simulink model "Control_test"  (R2014b)
settings: Solver=FixedStepDiscrete  StartTime=0.0  StopTime=Inf  FixedStep=0.001  RelTol=1e-3
PostLoadFcn:
  | , if any(exist('dsrtsu_mdlpostloadfcn', 'file') == [2, 3, 6]), try dsrtsu_mdlpostloadfcn('Execute', bdroot); catch fprintf('Error in PostLoadFcn (dsrtsu_mdlpostloadfcn) for model "%s":\n %s\n', bdroot, lasterr); end, end,
undefined symbols (not defined in the file or in its folder): dtLocal, slcm
libraries: rtican x163, simulink x14
(part 24 of 34)

== system Control_test/InputProcessing/RadarCanProcessing/Track34 ==
  Bus Creator : BusCreator  Inputs=12
  ESR_Track34 : rtican/RTICAN Receive (RX)   Reserved1=[]  Reserved2=[]  Reserved3=[]  Reserved4=[]  SfcnMessage=[]  Msg_Struct=[]  BoardTypeNo=[]  BoardNo=[]  ChannelNo=[]  Parameters=[]  DialogFcn=[]  UnitName=[]  Revision=[]  UnitValues=[]  DSProperties=struct('RTI',struct('Version',uint32(5),'BlockType',struct('isSLSource',uint8(1),'isSLSink',uint8(1),'isHWSource',uint8(0),'isHWSink',uint8(0),'isSetup',uint8(0),'isInline',uint8(1),'isNonInline',uint8(0),'isInterrupt',uint8(0),'isChannelwise',uint8(0)),'IOBoardType','RTICAN','UnitType','MESSAGE','Identifier','RX','DialogType','MSVC','BlockSet','RTICAN','SlaveProcessor','CAN'))  RTIBlockInterface=struct('OutputPortsWidth',int32([1 1 1 1 1 1 1 1 1 1 1 1]),'OutputPortsActive',[1 1 1 1 1 1 1 1 1 1 1 1],'OutputPortsName',{{'CAN_TX_TRACK_RANGE_RATE_34','CAN_TX_TRACK_MED_RANGE_MODE_34','CAN_TX_TRACK_RANGE_ACCEL_34','CAN_TX_TRACK_WIDTH_34','CAN_TX_TRACK_ROLLING_COUNT_34','CAN_TX_TRACK_BRIDGE_OBJECT_34','CAN_TX_TRACK_RANGE_34','CAN_TX_TRACK_ANGLE_34','CAN_TX_TRACK_STATUS_34','CAN_TX_TRACK_ONCOMING_34','CAN_TX_TRACK_GROUPING_CHANGED_34','CAN_TX_TRACK_LAT_RATE_34'}},'OutputPortsDataType',{{'SS_DOUBLE','SS_DOUBLE','SS_DOUBLE','SS_DOUBLE','SS_DOUBLE','SS_DOUBLE','SS_DOUBLE','SS_DOUBLE','SS_DOUBLE','SS_DOUBLE','SS_DOUBLE','SS_DOUBLE'}},'OutputPortsLabel',{{'CAN_TX_TRACK_RANGE_RATE_34','CAN_TX_TRACK_MED_RANGE_MODE_34','CAN_TX_TRACK_RANGE_ACCEL_34','CAN_TX_TRACK_WIDTH_34','CAN_TX_TRACK_ROLLING_COUNT_34','CAN_TX_TRACK_BRIDGE_OBJECT_34','CAN_TX_TRACK_RANGE_34','CAN_TX_TRACK_ANGLE_34','CAN_TX_TRACK_STATUS_34','CAN_TX_TRACK_ONCOMING_34','CAN_TX_TRACK_GROUPING_CHANGED_34','CAN_TX_TRACK_LAT_RATE_34'}},'OutputPortsLabelMode','ON','InputPortsWidth',int32(0),'InputPortsActive',0,'DialogFcn','rtican_message_interface_gui','BlockDisplay',{{'','center'}},'IconTransparency','on','ParameterTunableNames',{{}},'InitLevel',3,'BlockName',struct('Token',{{'ESR_Track34'}}),'SampleTime',{{0.01}},'TriggerPort',{{'none'}},'EnablePort',{{'none'}})  RTIBlockParameters=struct('BoardTypeNo',{{1,'OFF',[]}},'BoardNo',{{2,'ON',[1 16]}},'ChannelNo',{{2,'ON',[1 2]}},'Parameters',{{struct('DataFileSupport',struct('DataFileSelectedMaster',1,'DataFileSelectedLocal',0,'DataFileName','c:\users\mpc_car\documents\github\mpc-car\controller\dbcfiles\esr_dv3_64tgt.dbc|','DataFileDate',{{{['02-Nov-2012 20:32:52']},{['21-Mar-2013 13:39:53']},{['28-Sep-2011 17:08:52']}}},'SelectedFile',['<no file selected>'],'InterfaceFcn','rtican_dbc_file_parser'),'Options',struct('StatusSelected',0,'TimeSelected',0,'DeltaTimeSelected',0,'BytePortSelected',0,'MessageLengthSelected',0,'TriggerPort',struct('Selected',0,'TriggerType',0),'UserCoding',struct('Selected',0,'InterfaceFile','UserDecodingFile','FcnName','UserDecodeFcn','InportSelected',0,'InportWidth',1,'OutportSelected',0,'OutportWidth',1),'EnablePortSelected',0,'SignalOnPortnameSelected',1,'UseRXService',0),'Message',struct('MsgOnBlocknameSelected',1,'MsgName','ESR_Track34','MsgIdFormat',0,'MsgId',1313,'MsgLength',8,'NumSignals',12,'SampleTime',0.01,'Signal',struct('SgnName',{'CAN_TX_TRACK_RANGE_RATE_34','CAN_TX_TRACK_MED_RANGE_MODE_34','CAN_TX_TRACK_RANGE_ACCEL_34','CAN_TX_TRACK_WIDTH_34','CAN_TX_TRACK_ROLLING_COUNT_34','CAN_TX_TRACK_BRIDGE_OBJECT_34','CAN_TX_TRACK_RANGE_34','CAN_TX_TRACK_ANGLE_34','CAN_TX_TRACK_STATUS_34','CAN_TX_TRACK_ONCOMING_34','CAN_TX_TRACK_GROUPING_CHANGED_34','CAN_TX_TRACK_LAT_RATE_34'},'SgnStartBit',{0,14,16,26,30,31,32,43,53,56,57,58},'SgnLength',{14,2,10,4,1,1,11,10,3,1,1,6},'SgnType',{0,0,0,0,0,0,0,0,0,0,0,0},'ModeValue',{-1,-1,-1,-1,-1,-1,-1,-1,-1,-1,-1,-1},'DataType',{1,0,1,0,0,0,0,1,0,0,0,1},'ByteLayout',{2,2,2,2,2,2,2,2,2,2,2,2},'Factor',{0.01,1,0.05,0.5,1,1,0.1,0.1,1,1,1,0.25},'Offset',{0,0,0,0,0,0,0,0,0,0,0,0},'SgnComment',{{''},{''},{''},{''},{''},{''},{''},{''},{''},{''},{''},{''}},'SgnUnit',{'m/s','','m/s/s','m','','','m','deg','','','',''},'Min',{-81.92,0,-25.6,0,0,0,0,-51.2,0,0,0,-8},'Max',{81.91,3,25.55,7.5,1,0,204.7,51.1,7,0,0,7.75},'SLDataType',{'SS_DOUBLE','SS_DOUBLE','SS_DOUBLE','SS_DOUBLE','SS_DOUBLE','SS_DOUBLE','SS_DOUBLE','SS_DOUBLE','SS_DOUBLE','SS_DOUBLE','SS_DOUBLE','SS_DOUBLE'}),'MsgIdNumFormat',0,'MsgComment',{{''}}),'Version',1.2,'general',struct('isFromLib',0)),'OFF',[]}},'GroupId',{{struct('Group',{{'RTICAN'}},'No',4,'Behavior',{{'NAMECHANGE'}},'BlockType',{{'SINK'}},'NameChangeFlag',0),'OFF',[]}},'SFcnRTICANMessage',{{struct('MsgType','RX','SFcnPortType','Scalar','MsgName','ESR_Track34','MsgIdFormat','STD','MsgId',1313,'MsgLength',8,'NumSignals',12,'SampleTime',0.01,'Signal',struct('SgnName',{'CAN_TX_TRACK_RANGE_RATE_34','CAN_TX_TRACK_MED_RANGE_MODE_34','CAN_TX_TRACK_RANGE_ACCEL_34','CAN_TX_TRACK_WIDTH_34','CAN_TX_TRACK_ROLLING_COUNT_34','CAN_TX_TRACK_BRIDGE_OBJECT_34','CAN_TX_TRACK_RANGE_34','CAN_TX_TRACK_ANGLE_34','CAN_TX_TRACK_STATUS_34','CAN_TX_TRACK_ONCOMING_34','CAN_TX_TRACK_GROUPING_CHANGED_34','CAN_TX_TRACK_LAT_RATE_34'},'SgnStartBit',{0,14,16,26,30,31,32,43,53,56,57,58},'SgnLength',{14,2,10,4,1,1,11,10,3,1,1,6},'SgnType',{'standard','standard','standard','standard','standard','standard','standard','standard','standard','standard','standard','standard'},'ModeValue',{-1,-1,-1,-1,-1,-1,-1,-1,-1,-1,-1,-1},'DataType',{['signed int'],['unsigned int'],['signed int'],['unsigned int'],['unsigned int'],['unsigned int'],['unsigned int'],['signed int'],['unsigned int'],['unsigned int'],['unsigned int'],['signed int']},'ByteLayout',{['motorola back.'],['motorola back.'],['motorola back.'],['motorola back.'],['motorola back.'],['motorola back.'],['motorola back.'],['motorola back.'],['motorola back.'],['motorola back.'],['motorola back.'],['motorola back.']},'Factor',{0.01,1,0.05,0.5,1,1,0.1,0.1,1,1,1,0.25},'Offset',{0,0,0,0,0,0,0,0,0,0,0,0},'SLDataType',{'SS_DOUBLE','SS_DOUBLE','SS_DOUBLE','SS_DOUBLE','SS_DOUBLE','SS_DOUBLE','SS_DOUBLE','SS_DOUBLE','SS_DOUBLE','SS_DOUBLE','SS_DOUBLE','SS_DOUBLE'}),'StatusSelected','no','TimeSelected','no','DeltaTimeSelected','no','BytePortSelected','no','MessageLengthSelected','no','TriggerPort',struct('Selected','no','TriggerType',0),'UserCoding',struct('Selected','no','InterfaceFile','UserDecodingFile','FcnName','UserDecodeFcn','InportSelected','no','InportWidth',1,'OutportSelected','no','OutportWidth',1),'EnablePortSelected','no','UseRXService','no','BoardType','DS1','BoardNo',2,'ControllerNo',2),'OFF',[]}},'TLCFileName',{{'rtican_rx_message','OFF',[]}})  RTISFcnParameters=struct('SFcnRTICANMessage','struct','TLCFileName','char')  RTIBlockParaDefault=struct('BoardTypeNo',4302,'BoardNo',1,'ChannelNo',1,'Parameters',struct('DataFileSupport',struct('DataFileSelectedMaster',0,'DataFileSelectedLocal',0,'DataFileName','','DataFileDate','','SelectedFile',['<no file selected>']),'Options',struct('StatusSelected',1,'TimeSelected',1,'DeltaTimeSelected',1,'BytePortSelected',0,'MessageLengthSelected',0,'TriggerPort',struct('Selected',0,'TriggerType','rising'),'UserCoding',struct('Selected',0,'InterfaceFile','UserDecodingFile','FcnName','UserDecodeFcn','InportSelected',0,'InportWidth',1,'OutportSelected',0,'OutportWidth',1),'EnablePortSelected',0,'SignalOnPortnameSelected',1,'UseRXService',0),'Message',struct('MsgOnBlocknameSelected',0,'MsgName',['RX Message'],'MsgIdFormat',0,'MsgId',100,'MsgLength',8,'NumSignals',1,'SampleTime',-1,'Signal',struct('SgnName',['RX signal'],'SgnStartBit',0,'SgnLength',8,'SgnType',0,'ModeValue',-1,'DataType',0,'SLDataType','SS_DOUBLE','ByteLayout',0,'Factor',1,'Offset',0,'Min',0,'Max',255,'SgnComment',{{}},'SgnUnit',''),'MsgIdNumFormat',0,'MsgComment',{{''}}),'Version',1.2,'general',struct('isFromLib',1)),'GroupId',struct('Group',{{'RTICAN'}},'No',1,'Behavior',{{'NAMECHANGE'}},'BlockType',{{'SINK'}},'NameChangeFlag',0),'SFcnRTICANMessage',struct('MsgType','RX','MsgName',['RX Message'],'MsgIdFormat','STD','MsgId',100,'MsgLength',8,'NumSignals',1,'SampleTime',-1,'Signal',struct('SgnName',['RX signal'],'SgnStartBit',0,'SgnLength',8,'SgnType','standard','ModeValue',-1,'DataType',['unsigned int'],'ByteLayout',['little endian'],'SLDataType','SS_DOUBLE','Factor',1,'Offset',0),'StatusSelected','yes','TimeSelected','yes','DeltaTimeSelected','yes','BytePortSelected','no','MessageLengthSelected','no','EnablePortSelected','no','UserCoding',struct('Selected','no','InterfaceFile','UserDecodingFile','FcnName','UserDecodeFcn','InportSelected','no','InportWidth',1,'OutportSelected','no','OutportWidth',1),'TriggerPort',struct('Selected','no','TriggerType','rising'),'UseRXService','no','BoardType','DS4302','BoardNo',1,'ControllerNo',1,'SFcnPortType','Scalar'),'TLCFileName','rtican_rx_message')
      settings: AttributesFormatString=Group Id: RTICAN4\n
  Out1 : Outport
  wires:
  Bus Creator/1 -> Out1/1  "Track34"
  ESR_Track34/1 -> Bus Creator/1  "CAN_TX_TRACK_RANGE_RATE_34"
  ESR_Track34/2 -> Bus Creator/2  "CAN_TX_TRACK_MED_RANGE_MODE_34"
  ESR_Track34/3 -> Bus Creator/3  "CAN_TX_TRACK_RANGE_ACCEL_34"
  ESR_Track34/4 -> Bus Creator/4  "CAN_TX_TRACK_WIDTH_34"
  ESR_Track34/5 -> Bus Creator/5  "CAN_TX_TRACK_ROLLING_COUNT_34"
  ESR_Track34/6 -> Bus Creator/6  "CAN_TX_TRACK_BRIDGE_OBJECT_34"
  ESR_Track34/7 -> Bus Creator/7  "CAN_TX_TRACK_RANGE_34"
  ESR_Track34/8 -> Bus Creator/8  "CAN_TX_TRACK_ANGLE_34"
  ESR_Track34/9 -> Bus Creator/9  "CAN_TX_TRACK_STATUS_34"
  ESR_Track34/10 -> Bus Creator/10  "CAN_TX_TRACK_ONCOMING_34"
  ESR_Track34/11 -> Bus Creator/11  "CAN_TX_TRACK_GROUPING_CHANGED_34"
  ESR_Track34/12 -> Bus Creator/12  "CAN_TX_TRACK_LAT_RATE_34"

== system Control_test/InputProcessing/RadarCanProcessing/Track35 ==
  Bus Creator : BusCreator  Inputs=12
  ESR_Track35 : rtican/RTICAN Receive (RX)   Reserved1=[]  Reserved2=[]  Reserved3=[]  Reserved4=[]  SfcnMessage=[]  Msg_Struct=[]  BoardTypeNo=[]  BoardNo=[]  ChannelNo=[]  Parameters=[]  DialogFcn=[]  UnitName=[]  Revision=[]  UnitValues=[]  DSProperties=struct('RTI',struct('Version',uint32(5),'BlockType',struct('isSLSource',uint8(1),'isSLSink',uint8(1),'isHWSource',uint8(0),'isHWSink',uint8(0),'isSetup',uint8(0),'isInline',uint8(1),'isNonInline',uint8(0),'isInterrupt',uint8(0),'isChannelwise',uint8(0)),'IOBoardType','RTICAN','UnitType','MESSAGE','Identifier','RX','DialogType','MSVC','BlockSet','RTICAN','SlaveProcessor','CAN'))  RTIBlockInterface=struct('OutputPortsWidth',int32([1 1 1 1 1 1 1 1 1 1 1 1]),'OutputPortsActive',[1 1 1 1 1 1 1 1 1 1 1 1],'OutputPortsName',{{'CAN_TX_TRACK_RANGE_RATE_35','CAN_TX_TRACK_MED_RANGE_MODE_35','CAN_TX_TRACK_RANGE_ACCEL_35','CAN_TX_TRACK_WIDTH_35','CAN_TX_TRACK_ROLLING_COUNT_35','CAN_TX_TRACK_BRIDGE_OBJECT_35','CAN_TX_TRACK_RANGE_35','CAN_TX_TRACK_ANGLE_35','CAN_TX_TRACK_STATUS_35','CAN_TX_TRACK_ONCOMING_35','CAN_TX_TRACK_GROUPING_CHANGED_35','CAN_TX_TRACK_LAT_RATE_35'}},'OutputPortsDataType',{{'SS_DOUBLE','SS_DOUBLE','SS_DOUBLE','SS_DOUBLE','SS_DOUBLE','SS_DOUBLE','SS_DOUBLE','SS_DOUBLE','SS_DOUBLE','SS_DOUBLE','SS_DOUBLE','SS_DOUBLE'}},'OutputPortsLabel',{{'CAN_TX_TRACK_RANGE_RATE_35','CAN_TX_TRACK_MED_RANGE_MODE_35','CAN_TX_TRACK_RANGE_ACCEL_35','CAN_TX_TRACK_WIDTH_35','CAN_TX_TRACK_ROLLING_COUNT_35','CAN_TX_TRACK_BRIDGE_OBJECT_35','CAN_TX_TRACK_RANGE_35','CAN_TX_TRACK_ANGLE_35','CAN_TX_TRACK_STATUS_35','CAN_TX_TRACK_ONCOMING_35','CAN_TX_TRACK_GROUPING_CHANGED_35','CAN_TX_TRACK_LAT_RATE_35'}},'OutputPortsLabelMode','ON','InputPortsWidth',int32(0),'InputPortsActive',0,'DialogFcn','rtican_message_interface_gui','BlockDisplay',{{'','center'}},'IconTransparency','on','ParameterTunableNames',{{}},'InitLevel',3,'BlockName',struct('Token',{{'ESR_Track35'}}),'SampleTime',{{0.01}},'TriggerPort',{{'none'}},'EnablePort',{{'none'}})  RTIBlockParameters=struct('BoardTypeNo',{{1,'OFF',[]}},'BoardNo',{{2,'ON',[1 16]}},'ChannelNo',{{2,'ON',[1 2]}},'Parameters',{{struct('DataFileSupport',struct('DataFileSelectedMaster',1,'DataFileSelectedLocal',0,'DataFileName','c:\users\mpc_car\documents\github\mpc-car\controller\dbcfiles\esr_dv3_64tgt.dbc|','DataFileDate',{{{['02-Nov-2012 20:32:52']},{['21-Mar-2013 13:39:53']},{['28-Sep-2011 17:08:52']}}},'SelectedFile',['<no file selected>'],'InterfaceFcn','rtican_dbc_file_parser'),'Options',struct('StatusSelected',0,'TimeSelected',0,'DeltaTimeSelected',0,'BytePortSelected',0,'MessageLengthSelected',0,'TriggerPort',struct('Selected',0,'TriggerType',0),'UserCoding',struct('Selected',0,'InterfaceFile','UserDecodingFile','FcnName','UserDecodeFcn','InportSelected',0,'InportWidth',1,'OutportSelected',0,'OutportWidth',1),'EnablePortSelected',0,'SignalOnPortnameSelected',1,'UseRXService',0),'Message',struct('MsgOnBlocknameSelected',1,'MsgName','ESR_Track35','MsgIdFormat',0,'MsgId',1314,'MsgLength',8,'NumSignals',12,'SampleTime',0.01,'Signal',struct('SgnName',{'CAN_TX_TRACK_RANGE_RATE_35','CAN_TX_TRACK_MED_RANGE_MODE_35','CAN_TX_TRACK_RANGE_ACCEL_35','CAN_TX_TRACK_WIDTH_35','CAN_TX_TRACK_ROLLING_COUNT_35','CAN_TX_TRACK_BRIDGE_OBJECT_35','CAN_TX_TRACK_RANGE_35','CAN_TX_TRACK_ANGLE_35','CAN_TX_TRACK_STATUS_35','CAN_TX_TRACK_ONCOMING_35','CAN_TX_TRACK_GROUPING_CHANGED_35','CAN_TX_TRACK_LAT_RATE_35'},'SgnStartBit',{0,14,16,26,30,31,32,43,53,56,57,58},'SgnLength',{14,2,10,4,1,1,11,10,3,1,1,6},'SgnType',{0,0,0,0,0,0,0,0,0,0,0,0},'ModeValue',{-1,-1,-1,-1,-1,-1,-1,-1,-1,-1,-1,-1},'DataType',{1,0,1,0,0,0,0,1,0,0,0,1},'ByteLayout',{2,2,2,2,2,2,2,2,2,2,2,2},'Factor',{0.01,1,0.05,0.5,1,1,0.1,0.1,1,1,1,0.25},'Offset',{0,0,0,0,0,0,0,0,0,0,0,0},'SgnComment',{{''},{''},{''},{''},{''},{''},{''},{''},{''},{''},{''},{''}},'SgnUnit',{'m/s','','m/s/s','m','','','m','deg','','','',''},'Min',{-81.92,0,-25.6,0,0,0,0,-51.2,0,0,0,-8},'Max',{81.91,3,25.55,7.5,1,0,204.7,51.1,7,0,0,7.75},'SLDataType',{'SS_DOUBLE','SS_DOUBLE','SS_DOUBLE','SS_DOUBLE','SS_DOUBLE','SS_DOUBLE','SS_DOUBLE','SS_DOUBLE','SS_DOUBLE','SS_DOUBLE','SS_DOUBLE','SS_DOUBLE'}),'MsgIdNumFormat',0,'MsgComment',{{''}}),'Version',1.2,'general',struct('isFromLib',0)),'OFF',[]}},'GroupId',{{struct('Group',{{'RTICAN'}},'No',4,'Behavior',{{'NAMECHANGE'}},'BlockType',{{'SINK'}},'NameChangeFlag',0),'OFF',[]}},'SFcnRTICANMessage',{{struct('MsgType','RX','SFcnPortType','Scalar','MsgName','ESR_Track35','MsgIdFormat','STD','MsgId',1314,'MsgLength',8,'NumSignals',12,'SampleTime',0.01,'Signal',struct('SgnName',{'CAN_TX_TRACK_RANGE_RATE_35','CAN_TX_TRACK_MED_RANGE_MODE_35','CAN_TX_TRACK_RANGE_ACCEL_35','CAN_TX_TRACK_WIDTH_35','CAN_TX_TRACK_ROLLING_COUNT_35','CAN_TX_TRACK_BRIDGE_OBJECT_35','CAN_TX_TRACK_RANGE_35','CAN_TX_TRACK_ANGLE_35','CAN_TX_TRACK_STATUS_35','CAN_TX_TRACK_ONCOMING_35','CAN_TX_TRACK_GROUPING_CHANGED_35','CAN_TX_TRACK_LAT_RATE_35'},'SgnStartBit',{0,14,16,26,30,31,32,43,53,56,57,58},'SgnLength',{14,2,10,4,1,1,11,10,3,1,1,6},'SgnType',{'standard','standard','standard','standard','standard','standard','standard','standard','standard','standard','standard','standard'},'ModeValue',{-1,-1,-1,-1,-1,-1,-1,-1,-1,-1,-1,-1},'DataType',{['signed int'],['unsigned int'],['signed int'],['unsigned int'],['unsigned int'],['unsigned int'],['unsigned int'],['signed int'],['unsigned int'],['unsigned int'],['unsigned int'],['signed int']},'ByteLayout',{['motorola back.'],['motorola back.'],['motorola back.'],['motorola back.'],['motorola back.'],['motorola back.'],['motorola back.'],['motorola back.'],['motorola back.'],['motorola back.'],['motorola back.'],['motorola back.']},'Factor',{0.01,1,0.05,0.5,1,1,0.1,0.1,1,1,1,0.25},'Offset',{0,0,0,0,0,0,0,0,0,0,0,0},'SLDataType',{'SS_DOUBLE','SS_DOUBLE','SS_DOUBLE','SS_DOUBLE','SS_DOUBLE','SS_DOUBLE','SS_DOUBLE','SS_DOUBLE','SS_DOUBLE','SS_DOUBLE','SS_DOUBLE','SS_DOUBLE'}),'StatusSelected','no','TimeSelected','no','DeltaTimeSelected','no','BytePortSelected','no','MessageLengthSelected','no','TriggerPort',struct('Selected','no','TriggerType',0),'UserCoding',struct('Selected','no','InterfaceFile','UserDecodingFile','FcnName','UserDecodeFcn','InportSelected','no','InportWidth',1,'OutportSelected','no','OutportWidth',1),'EnablePortSelected','no','UseRXService','no','BoardType','DS1','BoardNo',2,'ControllerNo',2),'OFF',[]}},'TLCFileName',{{'rtican_rx_message','OFF',[]}})  RTISFcnParameters=struct('SFcnRTICANMessage','struct','TLCFileName','char')  RTIBlockParaDefault=struct('BoardTypeNo',4302,'BoardNo',1,'ChannelNo',1,'Parameters',struct('DataFileSupport',struct('DataFileSelectedMaster',0,'DataFileSelectedLocal',0,'DataFileName','','DataFileDate','','SelectedFile',['<no file selected>']),'Options',struct('StatusSelected',1,'TimeSelected',1,'DeltaTimeSelected',1,'BytePortSelected',0,'MessageLengthSelected',0,'TriggerPort',struct('Selected',0,'TriggerType','rising'),'UserCoding',struct('Selected',0,'InterfaceFile','UserDecodingFile','FcnName','UserDecodeFcn','InportSelected',0,'InportWidth',1,'OutportSelected',0,'OutportWidth',1),'EnablePortSelected',0,'SignalOnPortnameSelected',1,'UseRXService',0),'Message',struct('MsgOnBlocknameSelected',0,'MsgName',['RX Message'],'MsgIdFormat',0,'MsgId',100,'MsgLength',8,'NumSignals',1,'SampleTime',-1,'Signal',struct('SgnName',['RX signal'],'SgnStartBit',0,'SgnLength',8,'SgnType',0,'ModeValue',-1,'DataType',0,'SLDataType','SS_DOUBLE','ByteLayout',0,'Factor',1,'Offset',0,'Min',0,'Max',255,'SgnComment',{{}},'SgnUnit',''),'MsgIdNumFormat',0,'MsgComment',{{''}}),'Version',1.2,'general',struct('isFromLib',1)),'GroupId',struct('Group',{{'RTICAN'}},'No',1,'Behavior',{{'NAMECHANGE'}},'BlockType',{{'SINK'}},'NameChangeFlag',0),'SFcnRTICANMessage',struct('MsgType','RX','MsgName',['RX Message'],'MsgIdFormat','STD','MsgId',100,'MsgLength',8,'NumSignals',1,'SampleTime',-1,'Signal',struct('SgnName',['RX signal'],'SgnStartBit',0,'SgnLength',8,'SgnType','standard','ModeValue',-1,'DataType',['unsigned int'],'ByteLayout',['little endian'],'SLDataType','SS_DOUBLE','Factor',1,'Offset',0),'StatusSelected','yes','TimeSelected','yes','DeltaTimeSelected','yes','BytePortSelected','no','MessageLengthSelected','no','EnablePortSelected','no','UserCoding',struct('Selected','no','InterfaceFile','UserDecodingFile','FcnName','UserDecodeFcn','InportSelected','no','InportWidth',1,'OutportSelected','no','OutportWidth',1),'TriggerPort',struct('Selected','no','TriggerType','rising'),'UseRXService','no','BoardType','DS4302','BoardNo',1,'ControllerNo',1,'SFcnPortType','Scalar'),'TLCFileName','rtican_rx_message')
      settings: AttributesFormatString=Group Id: RTICAN4\n
  Out1 : Outport
  wires:
  Bus Creator/1 -> Out1/1  "Track35"
  ESR_Track35/1 -> Bus Creator/1  "CAN_TX_TRACK_RANGE_RATE_35"
  ESR_Track35/2 -> Bus Creator/2  "CAN_TX_TRACK_MED_RANGE_MODE_35"
  ESR_Track35/3 -> Bus Creator/3  "CAN_TX_TRACK_RANGE_ACCEL_35"
  ESR_Track35/4 -> Bus Creator/4  "CAN_TX_TRACK_WIDTH_35"
  ESR_Track35/5 -> Bus Creator/5  "CAN_TX_TRACK_ROLLING_COUNT_35"
  ESR_Track35/6 -> Bus Creator/6  "CAN_TX_TRACK_BRIDGE_OBJECT_35"
  ESR_Track35/7 -> Bus Creator/7  "CAN_TX_TRACK_RANGE_35"
  ESR_Track35/8 -> Bus Creator/8  "CAN_TX_TRACK_ANGLE_35"
  ESR_Track35/9 -> Bus Creator/9  "CAN_TX_TRACK_STATUS_35"
  ESR_Track35/10 -> Bus Creator/10  "CAN_TX_TRACK_ONCOMING_35"
  ESR_Track35/11 -> Bus Creator/11  "CAN_TX_TRACK_GROUPING_CHANGED_35"
  ESR_Track35/12 -> Bus Creator/12  "CAN_TX_TRACK_LAT_RATE_35"

== system Control_test/InputProcessing/RadarCanProcessing/Track36 ==
  Bus Creator : BusCreator  Inputs=12
  ESR_Track36 : rtican/RTICAN Receive (RX)   Reserved1=[]  Reserved2=[]  Reserved3=[]  Reserved4=[]  SfcnMessage=[]  Msg_Struct=[]  BoardTypeNo=[]  BoardNo=[]  ChannelNo=[]  Parameters=[]  DialogFcn=[]  UnitName=[]  Revision=[]  UnitValues=[]  DSProperties=struct('RTI',struct('Version',uint32(5),'BlockType',struct('isSLSource',uint8(1),'isSLSink',uint8(1),'isHWSource',uint8(0),'isHWSink',uint8(0),'isSetup',uint8(0),'isInline',uint8(1),'isNonInline',uint8(0),'isInterrupt',uint8(0),'isChannelwise',uint8(0)),'IOBoardType','RTICAN','UnitType','MESSAGE','Identifier','RX','DialogType','MSVC','BlockSet','RTICAN','SlaveProcessor','CAN'))  RTIBlockInterface=struct('OutputPortsWidth',int32([1 1 1 1 1 1 1 1 1 1 1 1]),'OutputPortsActive',[1 1 1 1 1 1 1 1 1 1 1 1],'OutputPortsName',{{'CAN_TX_TRACK_RANGE_RATE_36','CAN_TX_TRACK_MED_RANGE_MODE_36','CAN_TX_TRACK_RANGE_ACCEL_36','CAN_TX_TRACK_WIDTH_36','CAN_TX_TRACK_ROLLING_COUNT_36','CAN_TX_TRACK_BRIDGE_OBJECT_36','CAN_TX_TRACK_RANGE_36','CAN_TX_TRACK_ANGLE_36','CAN_TX_TRACK_STATUS_36','CAN_TX_TRACK_ONCOMING_36','CAN_TX_TRACK_GROUPING_CHANGED_36','CAN_TX_TRACK_LAT_RATE_36'}},'OutputPortsDataType',{{'SS_DOUBLE','SS_DOUBLE','SS_DOUBLE','SS_DOUBLE','SS_DOUBLE','SS_DOUBLE','SS_DOUBLE','SS_DOUBLE','SS_DOUBLE','SS_DOUBLE','SS_DOUBLE','SS_DOUBLE'}},'OutputPortsLabel',{{'CAN_TX_TRACK_RANGE_RATE_36','CAN_TX_TRACK_MED_RANGE_MODE_36','CAN_TX_TRACK_RANGE_ACCEL_36','CAN_TX_TRACK_WIDTH_36','CAN_TX_TRACK_ROLLING_COUNT_36','CAN_TX_TRACK_BRIDGE_OBJECT_36','CAN_TX_TRACK_RANGE_36','CAN_TX_TRACK_ANGLE_36','CAN_TX_TRACK_STATUS_36','CAN_TX_TRACK_ONCOMING_36','CAN_TX_TRACK_GROUPING_CHANGED_36','CAN_TX_TRACK_LAT_RATE_36'}},'OutputPortsLabelMode','ON','InputPortsWidth',int32(0),'InputPortsActive',0,'DialogFcn','rtican_message_interface_gui','BlockDisplay',{{'','center'}},'IconTransparency','on','ParameterTunableNames',{{}},'InitLevel',3,'BlockName',struct('Token',{{'ESR_Track36'}}),'SampleTime',{{0.01}},'TriggerPort',{{'none'}},'EnablePort',{{'none'}})  RTIBlockParameters=struct('BoardTypeNo',{{1,'OFF',[]}},'BoardNo',{{2,'ON',[1 16]}},'ChannelNo',{{2,'ON',[1 2]}},'Parameters',{{struct('DataFileSupport',struct('DataFileSelectedMaster',1,'DataFileSelectedLocal',0,'DataFileName','c:\users\mpc_car\documents\github\mpc-car\controller\dbcfiles\esr_dv3_64tgt.dbc|','DataFileDate',{{{['02-Nov-2012 20:32:52']},{['21-Mar-2013 13:39:53']},{['28-Sep-2011 17:08:52']}}},'SelectedFile',['<no file selected>'],'InterfaceFcn','rtican_dbc_file_parser'),'Options',struct('StatusSelected',0,'TimeSelected',0,'DeltaTimeSelected',0,'BytePortSelected',0,'MessageLengthSelected',0,'TriggerPort',struct('Selected',0,'TriggerType',0),'UserCoding',struct('Selected',0,'InterfaceFile','UserDecodingFile','FcnName','UserDecodeFcn','InportSelected',0,'InportWidth',1,'OutportSelected',0,'OutportWidth',1),'EnablePortSelected',0,'SignalOnPortnameSelected',1,'UseRXService',0),'Message',struct('MsgOnBlocknameSelected',1,'MsgName','ESR_Track36','MsgIdFormat',0,'MsgId',1315,'MsgLength',8,'NumSignals',12,'SampleTime',0.01,'Signal',struct('SgnName',{'CAN_TX_TRACK_RANGE_RATE_36','CAN_TX_TRACK_MED_RANGE_MODE_36','CAN_TX_TRACK_RANGE_ACCEL_36','CAN_TX_TRACK_WIDTH_36','CAN_TX_TRACK_ROLLING_COUNT_36','CAN_TX_TRACK_BRIDGE_OBJECT_36','CAN_TX_TRACK_RANGE_36','CAN_TX_TRACK_ANGLE_36','CAN_TX_TRACK_STATUS_36','CAN_TX_TRACK_ONCOMING_36','CAN_TX_TRACK_GROUPING_CHANGED_36','CAN_TX_TRACK_LAT_RATE_36'},'SgnStartBit',{0,14,16,26,30,31,32,43,53,56,57,58},'SgnLength',{14,2,10,4,1,1,11,10,3,1,1,6},'SgnType',{0,0,0,0,0,0,0,0,0,0,0,0},'ModeValue',{-1,-1,-1,-1,-1,-1,-1,-1,-1,-1,-1,-1},'DataType',{1,0,1,0,0,0,0,1,0,0,0,1},'ByteLayout',{2,2,2,2,2,2,2,2,2,2,2,2},'Factor',{0.01,1,0.05,0.5,1,1,0.1,0.1,1,1,1,0.25},'Offset',{0,0,0,0,0,0,0,0,0,0,0,0},'SgnComment',{{''},{''},{''},{''},{''},{''},{''},{''},{''},{''},{''},{''}},'SgnUnit',{'m/s','','m/s/s','m','','','m','deg','','','',''},'Min',{-81.92,0,-25.6,0,0,0,0,-51.2,0,0,0,-8},'Max',{81.91,3,25.55,7.5,1,0,204.7,51.1,7,0,0,7.75},'SLDataType',{'SS_DOUBLE','SS_DOUBLE','SS_DOUBLE','SS_DOUBLE','SS_DOUBLE','SS_DOUBLE','SS_DOUBLE','SS_DOUBLE','SS_DOUBLE','SS_DOUBLE','SS_DOUBLE','SS_DOUBLE'}),'MsgIdNumFormat',0,'MsgComment',{{''}}),'Version',1.2,'general',struct('isFromLib',0)),'OFF',[]}},'GroupId',{{struct('Group',{{'RTICAN'}},'No',4,'Behavior',{{'NAMECHANGE'}},'BlockType',{{'SINK'}},'NameChangeFlag',0),'OFF',[]}},'SFcnRTICANMessage',{{struct('MsgType','RX','SFcnPortType','Scalar','MsgName','ESR_Track36','MsgIdFormat','STD','MsgId',1315,'MsgLength',8,'NumSignals',12,'SampleTime',0.01,'Signal',struct('SgnName',{'CAN_TX_TRACK_RANGE_RATE_36','CAN_TX_TRACK_MED_RANGE_MODE_36','CAN_TX_TRACK_RANGE_ACCEL_36','CAN_TX_TRACK_WIDTH_36','CAN_TX_TRACK_ROLLING_COUNT_36','CAN_TX_TRACK_BRIDGE_OBJECT_36','CAN_TX_TRACK_RANGE_36','CAN_TX_TRACK_ANGLE_36','CAN_TX_TRACK_STATUS_36','CAN_TX_TRACK_ONCOMING_36','CAN_TX_TRACK_GROUPING_CHANGED_36','CAN_TX_TRACK_LAT_RATE_36'},'SgnStartBit',{0,14,16,26,30,31,32,43,53,56,57,58},'SgnLength',{14,2,10,4,1,1,11,10,3,1,1,6},'SgnType',{'standard','standard','standard','standard','standard','standard','standard','standard','standard','standard','standard','standard'},'ModeValue',{-1,-1,-1,-1,-1,-1,-1,-1,-1,-1,-1,-1},'DataType',{['signed int'],['unsigned int'],['signed int'],['unsigned int'],['unsigned int'],['unsigned int'],['unsigned int'],['signed int'],['unsigned int'],['unsigned int'],['unsigned int'],['signed int']},'ByteLayout',{['motorola back.'],['motorola back.'],['motorola back.'],['motorola back.'],['motorola back.'],['motorola back.'],['motorola back.'],['motorola back.'],['motorola back.'],['motorola back.'],['motorola back.'],['motorola back.']},'Factor',{0.01,1,0.05,0.5,1,1,0.1,0.1,1,1,1,0.25},'Offset',{0,0,0,0,0,0,0,0,0,0,0,0},'SLDataType',{'SS_DOUBLE','SS_DOUBLE','SS_DOUBLE','SS_DOUBLE','SS_DOUBLE','SS_DOUBLE','SS_DOUBLE','SS_DOUBLE','SS_DOUBLE','SS_DOUBLE','SS_DOUBLE','SS_DOUBLE'}),'StatusSelected','no','TimeSelected','no','DeltaTimeSelected','no','BytePortSelected','no','MessageLengthSelected','no','TriggerPort',struct('Selected','no','TriggerType',0),'UserCoding',struct('Selected','no','InterfaceFile','UserDecodingFile','FcnName','UserDecodeFcn','InportSelected','no','InportWidth',1,'OutportSelected','no','OutportWidth',1),'EnablePortSelected','no','UseRXService','no','BoardType','DS1','BoardNo',2,'ControllerNo',2),'OFF',[]}},'TLCFileName',{{'rtican_rx_message','OFF',[]}})  RTISFcnParameters=struct('SFcnRTICANMessage','struct','TLCFileName','char')  RTIBlockParaDefault=struct('BoardTypeNo',4302,'BoardNo',1,'ChannelNo',1,'Parameters',struct('DataFileSupport',struct('DataFileSelectedMaster',0,'DataFileSelectedLocal',0,'DataFileName','','DataFileDate','','SelectedFile',['<no file selected>']),'Options',struct('StatusSelected',1,'TimeSelected',1,'DeltaTimeSelected',1,'BytePortSelected',0,'MessageLengthSelected',0,'TriggerPort',struct('Selected',0,'TriggerType','rising'),'UserCoding',struct('Selected',0,'InterfaceFile','UserDecodingFile','FcnName','UserDecodeFcn','InportSelected',0,'InportWidth',1,'OutportSelected',0,'OutportWidth',1),'EnablePortSelected',0,'SignalOnPortnameSelected',1,'UseRXService',0),'Message',struct('MsgOnBlocknameSelected',0,'MsgName',['RX Message'],'MsgIdFormat',0,'MsgId',100,'MsgLength',8,'NumSignals',1,'SampleTime',-1,'Signal',struct('SgnName',['RX signal'],'SgnStartBit',0,'SgnLength',8,'SgnType',0,'ModeValue',-1,'DataType',0,'SLDataType','SS_DOUBLE','ByteLayout',0,'Factor',1,'Offset',0,'Min',0,'Max',255,'SgnComment',{{}},'SgnUnit',''),'MsgIdNumFormat',0,'MsgComment',{{''}}),'Version',1.2,'general',struct('isFromLib',1)),'GroupId',struct('Group',{{'RTICAN'}},'No',1,'Behavior',{{'NAMECHANGE'}},'BlockType',{{'SINK'}},'NameChangeFlag',0),'SFcnRTICANMessage',struct('MsgType','RX','MsgName',['RX Message'],'MsgIdFormat','STD','MsgId',100,'MsgLength',8,'NumSignals',1,'SampleTime',-1,'Signal',struct('SgnName',['RX signal'],'SgnStartBit',0,'SgnLength',8,'SgnType','standard','ModeValue',-1,'DataType',['unsigned int'],'ByteLayout',['little endian'],'SLDataType','SS_DOUBLE','Factor',1,'Offset',0),'StatusSelected','yes','TimeSelected','yes','DeltaTimeSelected','yes','BytePortSelected','no','MessageLengthSelected','no','EnablePortSelected','no','UserCoding',struct('Selected','no','InterfaceFile','UserDecodingFile','FcnName','UserDecodeFcn','InportSelected','no','InportWidth',1,'OutportSelected','no','OutportWidth',1),'TriggerPort',struct('Selected','no','TriggerType','rising'),'UseRXService','no','BoardType','DS4302','BoardNo',1,'ControllerNo',1,'SFcnPortType','Scalar'),'TLCFileName','rtican_rx_message')
      settings: AttributesFormatString=Group Id: RTICAN4\n
  Out1 : Outport
  wires:
  Bus Creator/1 -> Out1/1  "Track36"
  ESR_Track36/1 -> Bus Creator/1  "CAN_TX_TRACK_RANGE_RATE_36"
  ESR_Track36/2 -> Bus Creator/2  "CAN_TX_TRACK_MED_RANGE_MODE_36"
  ESR_Track36/3 -> Bus Creator/3  "CAN_TX_TRACK_RANGE_ACCEL_36"
  ESR_Track36/4 -> Bus Creator/4  "CAN_TX_TRACK_WIDTH_36"
  ESR_Track36/5 -> Bus Creator/5  "CAN_TX_TRACK_ROLLING_COUNT_36"
  ESR_Track36/6 -> Bus Creator/6  "CAN_TX_TRACK_BRIDGE_OBJECT_36"
  ESR_Track36/7 -> Bus Creator/7  "CAN_TX_TRACK_RANGE_36"
  ESR_Track36/8 -> Bus Creator/8  "CAN_TX_TRACK_ANGLE_36"
  ESR_Track36/9 -> Bus Creator/9  "CAN_TX_TRACK_STATUS_36"
  ESR_Track36/10 -> Bus Creator/10  "CAN_TX_TRACK_ONCOMING_36"
  ESR_Track36/11 -> Bus Creator/11  "CAN_TX_TRACK_GROUPING_CHANGED_36"
  ESR_Track36/12 -> Bus Creator/12  "CAN_TX_TRACK_LAT_RATE_36"

== system Control_test/InputProcessing/RadarCanProcessing/Track37 ==
  Bus Creator : BusCreator  Inputs=12
  ESR_Track37 : rtican/RTICAN Receive (RX)   Reserved1=[]  Reserved2=[]  Reserved3=[]  Reserved4=[]  SfcnMessage=[]  Msg_Struct=[]  BoardTypeNo=[]  BoardNo=[]  ChannelNo=[]  Parameters=[]  DialogFcn=[]  UnitName=[]  Revision=[]  UnitValues=[]  DSProperties=struct('RTI',struct('Version',uint32(5),'BlockType',struct('isSLSource',uint8(1),'isSLSink',uint8(1),'isHWSource',uint8(0),'isHWSink',uint8(0),'isSetup',uint8(0),'isInline',uint8(1),'isNonInline',uint8(0),'isInterrupt',uint8(0),'isChannelwise',uint8(0)),'IOBoardType','RTICAN','UnitType','MESSAGE','Identifier','RX','DialogType','MSVC','BlockSet','RTICAN','SlaveProcessor','CAN'))  RTIBlockInterface=struct('OutputPortsWidth',int32([1 1 1 1 1 1 1 1 1 1 1 1]),'OutputPortsActive',[1 1 1 1 1 1 1 1 1 1 1 1],'OutputPortsName',{{'CAN_TX_TRACK_RANGE_RATE_37','CAN_TX_TRACK_MED_RANGE_MODE_37','CAN_TX_TRACK_RANGE_ACCEL_37','CAN_TX_TRACK_WIDTH_37','CAN_TX_TRACK_ROLLING_COUNT_37','CAN_TX_TRACK_BRIDGE_OBJECT_37','CAN_TX_TRACK_RANGE_37','CAN_TX_TRACK_ANGLE_37','CAN_TX_TRACK_STATUS_37','CAN_TX_TRACK_ONCOMING_37','CAN_TX_TRACK_GROUPING_CHANGED_37','CAN_TX_TRACK_LAT_RATE_37'}},'OutputPortsDataType',{{'SS_DOUBLE','SS_DOUBLE','SS_DOUBLE','SS_DOUBLE','SS_DOUBLE','SS_DOUBLE','SS_DOUBLE','SS_DOUBLE','SS_DOUBLE','SS_DOUBLE','SS_DOUBLE','SS_DOUBLE'}},'OutputPortsLabel',{{'CAN_TX_TRACK_RANGE_RATE_37','CAN_TX_TRACK_MED_RANGE_MODE_37','CAN_TX_TRACK_RANGE_ACCEL_37','CAN_TX_TRACK_WIDTH_37','CAN_TX_TRACK_ROLLING_COUNT_37','CAN_TX_TRACK_BRIDGE_OBJECT_37','CAN_TX_TRACK_RANGE_37','CAN_TX_TRACK_ANGLE_37','CAN_TX_TRACK_STATUS_37','CAN_TX_TRACK_ONCOMING_37','CAN_TX_TRACK_GROUPING_CHANGED_37','CAN_TX_TRACK_LAT_RATE_37'}},'OutputPortsLabelMode','ON','InputPortsWidth',int32(0),'InputPortsActive',0,'DialogFcn','rtican_message_interface_gui','BlockDisplay',{{'','center'}},'IconTransparency','on','ParameterTunableNames',{{}},'InitLevel',3,'BlockName',struct('Token',{{'ESR_Track37'}}),'SampleTime',{{0.01}},'TriggerPort',{{'none'}},'EnablePort',{{'none'}})  RTIBlockParameters=struct('BoardTypeNo',{{1,'OFF',[]}},'BoardNo',{{2,'ON',[1 16]}},'ChannelNo',{{2,'ON',[1 2]}},'Parameters',{{struct('DataFileSupport',struct('DataFileSelectedMaster',1,'DataFileSelectedLocal',0,'DataFileName','c:\users\mpc_car\documents\github\mpc-car\controller\dbcfiles\esr_dv3_64tgt.dbc|','DataFileDate',{{{['02-Nov-2012 20:32:52']},{['21-Mar-2013 13:39:53']},{['28-Sep-2011 17:08:52']}}},'SelectedFile',['<no file selected>'],'InterfaceFcn','rtican_dbc_file_parser'),'Options',struct('StatusSelected',0,'TimeSelected',0,'DeltaTimeSelected',0,'BytePortSelected',0,'MessageLengthSelected',0,'TriggerPort',struct('Selected',0,'TriggerType',0),'UserCoding',struct('Selected',0,'InterfaceFile','UserDecodingFile','FcnName','UserDecodeFcn','InportSelected',0,'InportWidth',1,'OutportSelected',0,'OutportWidth',1),'EnablePortSelected',0,'SignalOnPortnameSelected',1,'UseRXService',0),'Message',struct('MsgOnBlocknameSelected',1,'MsgName','ESR_Track37','MsgIdFormat',0,'MsgId',1316,'MsgLength',8,'NumSignals',12,'SampleTime',0.01,'Signal',struct('SgnName',{'CAN_TX_TRACK_RANGE_RATE_37','CAN_TX_TRACK_MED_RANGE_MODE_37','CAN_TX_TRACK_RANGE_ACCEL_37','CAN_TX_TRACK_WIDTH_37','CAN_TX_TRACK_ROLLING_COUNT_37','CAN_TX_TRACK_BRIDGE_OBJECT_37','CAN_TX_TRACK_RANGE_37','CAN_TX_TRACK_ANGLE_37','CAN_TX_TRACK_STATUS_37','CAN_TX_TRACK_ONCOMING_37','CAN_TX_TRACK_GROUPING_CHANGED_37','CAN_TX_TRACK_LAT_RATE_37'},'SgnStartBit',{0,14,16,26,30,31,32,43,53,56,57,58},'SgnLength',{14,2,10,4,1,1,11,10,3,1,1,6},'SgnType',{0,0,0,0,0,0,0,0,0,0,0,0},'ModeValue',{-1,-1,-1,-1,-1,-1,-1,-1,-1,-1,-1,-1},'DataType',{1,0,1,0,0,0,0,1,0,0,0,1},'ByteLayout',{2,2,2,2,2,2,2,2,2,2,2,2},'Factor',{0.01,1,0.05,0.5,1,1,0.1,0.1,1,1,1,0.25},'Offset',{0,0,0,0,0,0,0,0,0,0,0,0},'SgnComment',{{''},{''},{''},{''},{''},{''},{''},{''},{''},{''},{''},{''}},'SgnUnit',{'m/s','','m/s/s','m','','','m','deg','','','',''},'Min',{-81.92,0,-25.6,0,0,0,0,-51.2,0,0,0,-8},'Max',{81.91,3,25.55,7.5,1,0,204.7,51.1,7,0,0,7.75},'SLDataType',{'SS_DOUBLE','SS_DOUBLE','SS_DOUBLE','SS_DOUBLE','SS_DOUBLE','SS_DOUBLE','SS_DOUBLE','SS_DOUBLE','SS_DOUBLE','SS_DOUBLE','SS_DOUBLE','SS_DOUBLE'}),'MsgIdNumFormat',0,'MsgComment',{{''}}),'Version',1.2,'general',struct('isFromLib',0)),'OFF',[]}},'GroupId',{{struct('Group',{{'RTICAN'}},'No',4,'Behavior',{{'NAMECHANGE'}},'BlockType',{{'SINK'}},'NameChangeFlag',0),'OFF',[]}},'SFcnRTICANMessage',{{struct('MsgType','RX','SFcnPortType','Scalar','MsgName','ESR_Track37','MsgIdFormat','STD','MsgId',1316,'MsgLength',8,'NumSignals',12,'SampleTime',0.01,'Signal',struct('SgnName',{'CAN_TX_TRACK_RANGE_RATE_37','CAN_TX_TRACK_MED_RANGE_MODE_37','CAN_TX_TRACK_RANGE_ACCEL_37','CAN_TX_TRACK_WIDTH_37','CAN_TX_TRACK_ROLLING_COUNT_37','CAN_TX_TRACK_BRIDGE_OBJECT_37','CAN_TX_TRACK_RANGE_37','CAN_TX_TRACK_ANGLE_37','CAN_TX_TRACK_STATUS_37','CAN_TX_TRACK_ONCOMING_37','CAN_TX_TRACK_GROUPING_CHANGED_37','CAN_TX_TRACK_LAT_RATE_37'},'SgnStartBit',{0,14,16,26,30,31,32,43,53,56,57,58},'SgnLength',{14,2,10,4,1,1,11,10,3,1,1,6},'SgnType',{'standard','standard','standard','standard','standard','standard','standard','standard','standard','standard','standard','standard'},'ModeValue',{-1,-1,-1,-1,-1,-1,-1,-1,-1,-1,-1,-1},'DataType',{['signed int'],['unsigned int'],['signed int'],['unsigned int'],['unsigned int'],['unsigned int'],['unsigned int'],['signed int'],['unsigned int'],['unsigned int'],['unsigned int'],['signed int']},'ByteLayout',{['motorola back.'],['motorola back.'],['motorola back.'],['motorola back.'],['motorola back.'],['motorola back.'],['motorola back.'],['motorola back.'],['motorola back.'],['motorola back.'],['motorola back.'],['motorola back.']},'Factor',{0.01,1,0.05,0.5,1,1,0.1,0.1,1,1,1,0.25},'Offset',{0,0,0,0,0,0,0,0,0,0,0,0},'SLDataType',{'SS_DOUBLE','SS_DOUBLE','SS_DOUBLE','SS_DOUBLE','SS_DOUBLE','SS_DOUBLE','SS_DOUBLE','SS_DOUBLE','SS_DOUBLE','SS_DOUBLE','SS_DOUBLE','SS_DOUBLE'}),'StatusSelected','no','TimeSelected','no','DeltaTimeSelected','no','BytePortSelected','no','MessageLengthSelected','no','TriggerPort',struct('Selected','no','TriggerType',0),'UserCoding',struct('Selected','no','InterfaceFile','UserDecodingFile','FcnName','UserDecodeFcn','InportSelected','no','InportWidth',1,'OutportSelected','no','OutportWidth',1),'EnablePortSelected','no','UseRXService','no','BoardType','DS1','BoardNo',2,'ControllerNo',2),'OFF',[]}},'TLCFileName',{{'rtican_rx_message','OFF',[]}})  RTISFcnParameters=struct('SFcnRTICANMessage','struct','TLCFileName','char')  RTIBlockParaDefault=struct('BoardTypeNo',4302,'BoardNo',1,'ChannelNo',1,'Parameters',struct('DataFileSupport',struct('DataFileSelectedMaster',0,'DataFileSelectedLocal',0,'DataFileName','','DataFileDate','','SelectedFile',['<no file selected>']),'Options',struct('StatusSelected',1,'TimeSelected',1,'DeltaTimeSelected',1,'BytePortSelected',0,'MessageLengthSelected',0,'TriggerPort',struct('Selected',0,'TriggerType','rising'),'UserCoding',struct('Selected',0,'InterfaceFile','UserDecodingFile','FcnName','UserDecodeFcn','InportSelected',0,'InportWidth',1,'OutportSelected',0,'OutportWidth',1),'EnablePortSelected',0,'SignalOnPortnameSelected',1,'UseRXService',0),'Message',struct('MsgOnBlocknameSelected',0,'MsgName',['RX Message'],'MsgIdFormat',0,'MsgId',100,'MsgLength',8,'NumSignals',1,'SampleTime',-1,'Signal',struct('SgnName',['RX signal'],'SgnStartBit',0,'SgnLength',8,'SgnType',0,'ModeValue',-1,'DataType',0,'SLDataType','SS_DOUBLE','ByteLayout',0,'Factor',1,'Offset',0,'Min',0,'Max',255,'SgnComment',{{}},'SgnUnit',''),'MsgIdNumFormat',0,'MsgComment',{{''}}),'Version',1.2,'general',struct('isFromLib',1)),'GroupId',struct('Group',{{'RTICAN'}},'No',1,'Behavior',{{'NAMECHANGE'}},'BlockType',{{'SINK'}},'NameChangeFlag',0),'SFcnRTICANMessage',struct('MsgType','RX','MsgName',['RX Message'],'MsgIdFormat','STD','MsgId',100,'MsgLength',8,'NumSignals',1,'SampleTime',-1,'Signal',struct('SgnName',['RX signal'],'SgnStartBit',0,'SgnLength',8,'SgnType','standard','ModeValue',-1,'DataType',['unsigned int'],'ByteLayout',['little endian'],'SLDataType','SS_DOUBLE','Factor',1,'Offset',0),'StatusSelected','yes','TimeSelected','yes','DeltaTimeSelected','yes','BytePortSelected','no','MessageLengthSelected','no','EnablePortSelected','no','UserCoding',struct('Selected','no','InterfaceFile','UserDecodingFile','FcnName','UserDecodeFcn','InportSelected','no','InportWidth',1,'OutportSelected','no','OutportWidth',1),'TriggerPort',struct('Selected','no','TriggerType','rising'),'UseRXService','no','BoardType','DS4302','BoardNo',1,'ControllerNo',1,'SFcnPortType','Scalar'),'TLCFileName','rtican_rx_message')
      settings: AttributesFormatString=Group Id: RTICAN4\n
  Out1 : Outport
  wires:
  Bus Creator/1 -> Out1/1  "Track37"
  ESR_Track37/1 -> Bus Creator/1  "CAN_TX_TRACK_RANGE_RATE_37"
  ESR_Track37/2 -> Bus Creator/2  "CAN_TX_TRACK_MED_RANGE_MODE_37"
  ESR_Track37/3 -> Bus Creator/3  "CAN_TX_TRACK_RANGE_ACCEL_37"
  ESR_Track37/4 -> Bus Creator/4  "CAN_TX_TRACK_WIDTH_37"
  ESR_Track37/5 -> Bus Creator/5  "CAN_TX_TRACK_ROLLING_COUNT_37"
  ESR_Track37/6 -> Bus Creator/6  "CAN_TX_TRACK_BRIDGE_OBJECT_37"
  ESR_Track37/7 -> Bus Creator/7  "CAN_TX_TRACK_RANGE_37"
  ESR_Track37/8 -> Bus Creator/8  "CAN_TX_TRACK_ANGLE_37"
  ESR_Track37/9 -> Bus Creator/9  "CAN_TX_TRACK_STATUS_37"
  ESR_Track37/10 -> Bus Creator/10  "CAN_TX_TRACK_ONCOMING_37"
  ESR_Track37/11 -> Bus Creator/11  "CAN_TX_TRACK_GROUPING_CHANGED_37"
  ESR_Track37/12 -> Bus Creator/12  "CAN_TX_TRACK_LAT_RATE_37"

== system Control_test/InputProcessing/RadarCanProcessing/Track38 ==
  Bus Creator : BusCreator  Inputs=12
  ESR_Track38 : rtican/RTICAN Receive (RX)   Reserved1=[]  Reserved2=[]  Reserved3=[]  Reserved4=[]  SfcnMessage=[]  Msg_Struct=[]  BoardTypeNo=[]  BoardNo=[]  ChannelNo=[]  Parameters=[]  DialogFcn=[]  UnitName=[]  Revision=[]  UnitValues=[]  DSProperties=struct('RTI',struct('Version',uint32(5),'BlockType',struct('isSLSource',uint8(1),'isSLSink',uint8(1),'isHWSource',uint8(0),'isHWSink',uint8(0),'isSetup',uint8(0),'isInline',uint8(1),'isNonInline',uint8(0),'isInterrupt',uint8(0),'isChannelwise',uint8(0)),'IOBoardType','RTICAN','UnitType','MESSAGE','Identifier','RX','DialogType','MSVC','BlockSet','RTICAN','SlaveProcessor','CAN'))  RTIBlockInterface=struct('OutputPortsWidth',int32([1 1 1 1 1 1 1 1 1 1 1 1]),'OutputPortsActive',[1 1 1 1 1 1 1 1 1 1 1 1],'OutputPortsName',{{'CAN_TX_TRACK_RANGE_RATE_38','CAN_TX_TRACK_MED_RANGE_MODE_38','CAN_TX_TRACK_RANGE_ACCEL_38','CAN_TX_TRACK_WIDTH_38','CAN_TX_TRACK_ROLLING_COUNT_38','CAN_TX_TRACK_BRIDGE_OBJECT_38','CAN_TX_TRACK_RANGE_38','CAN_TX_TRACK_ANGLE_38','CAN_TX_TRACK_STATUS_38','CAN_TX_TRACK_ONCOMING_38','CAN_TX_TRACK_GROUPING_CHANGED_38','CAN_TX_TRACK_LAT_RATE_38'}},'OutputPortsDataType',{{'SS_DOUBLE','SS_DOUBLE','SS_DOUBLE','SS_DOUBLE','SS_DOUBLE','SS_DOUBLE','SS_DOUBLE','SS_DOUBLE','SS_DOUBLE','SS_DOUBLE','SS_DOUBLE','SS_DOUBLE'}},'OutputPortsLabel',{{'CAN_TX_TRACK_RANGE_RATE_38','CAN_TX_TRACK_MED_RANGE_MODE_38','CAN_TX_TRACK_RANGE_ACCEL_38','CAN_TX_TRACK_WIDTH_38','CAN_TX_TRACK_ROLLING_COUNT_38','CAN_TX_TRACK_BRIDGE_OBJECT_38','CAN_TX_TRACK_RANGE_38','CAN_TX_TRACK_ANGLE_38','CAN_TX_TRACK_STATUS_38','CAN_TX_TRACK_ONCOMING_38','CAN_TX_TRACK_GROUPING_CHANGED_38','CAN_TX_TRACK_LAT_RATE_38'}},'OutputPortsLabelMode','ON','InputPortsWidth',int32(0),'InputPortsActive',0,'DialogFcn','rtican_message_interface_gui','BlockDisplay',{{'','center'}},'IconTransparency','on','ParameterTunableNames',{{}},'InitLevel',3,'BlockName',struct('Token',{{'ESR_Track38'}}),'SampleTime',{{0.01}},'TriggerPort',{{'none'}},'EnablePort',{{'none'}})  RTIBlockParameters=struct('BoardTypeNo',{{1,'OFF',[]}},'BoardNo',{{2,'ON',[1 16]}},'ChannelNo',{{2,'ON',[1 2]}},'Parameters',{{struct('DataFileSupport',struct('DataFileSelectedMaster',1,'DataFileSelectedLocal',0,'DataFileName','c:\users\mpc_car\documents\github\mpc-car\controller\dbcfiles\esr_dv3_64tgt.dbc|','DataFileDate',{{{['02-Nov-2012 20:32:52']},{['21-Mar-2013 13:39:53']},{['28-Sep-2011 17:08:52']}}},'SelectedFile',['<no file selected>'],'InterfaceFcn','rtican_dbc_file_parser'),'Options',struct('StatusSelected',0,'TimeSelected',0,'DeltaTimeSelected',0,'BytePortSelected',0,'MessageLengthSelected',0,'TriggerPort',struct('Selected',0,'TriggerType',0),'UserCoding',struct('Selected',0,'InterfaceFile','UserDecodingFile','FcnName','UserDecodeFcn','InportSelected',0,'InportWidth',1,'OutportSelected',0,'OutportWidth',1),'EnablePortSelected',0,'SignalOnPortnameSelected',1,'UseRXService',0),'Message',struct('MsgOnBlocknameSelected',1,'MsgName','ESR_Track38','MsgIdFormat',0,'MsgId',1317,'MsgLength',8,'NumSignals',12,'SampleTime',0.01,'Signal',struct('SgnName',{'CAN_TX_TRACK_RANGE_RATE_38','CAN_TX_TRACK_MED_RANGE_MODE_38','CAN_TX_TRACK_RANGE_ACCEL_38','CAN_TX_TRACK_WIDTH_38','CAN_TX_TRACK_ROLLING_COUNT_38','CAN_TX_TRACK_BRIDGE_OBJECT_38','CAN_TX_TRACK_RANGE_38','CAN_TX_TRACK_ANGLE_38','CAN_TX_TRACK_STATUS_38','CAN_TX_TRACK_ONCOMING_38','CAN_TX_TRACK_GROUPING_CHANGED_38','CAN_TX_TRACK_LAT_RATE_38'},'SgnStartBit',{0,14,16,26,30,31,32,43,53,56,57,58},'SgnLength',{14,2,10,4,1,1,11,10,3,1,1,6},'SgnType',{0,0,0,0,0,0,0,0,0,0,0,0},'ModeValue',{-1,-1,-1,-1,-1,-1,-1,-1,-1,-1,-1,-1},'DataType',{1,0,1,0,0,0,0,1,0,0,0,1},'ByteLayout',{2,2,2,2,2,2,2,2,2,2,2,2},'Factor',{0.01,1,0.05,0.5,1,1,0.1,0.1,1,1,1,0.25},'Offset',{0,0,0,0,0,0,0,0,0,0,0,0},'SgnComment',{{''},{''},{''},{''},{''},{''},{''},{''},{''},{''},{''},{''}},'SgnUnit',{'m/s','','m/s/s','m','','','m','deg','','','',''},'Min',{-81.92,0,-25.6,0,0,0,0,-51.2,0,0,0,-8},'Max',{81.91,3,25.55,7.5,1,0,204.7,51.1,7,0,0,7.75},'SLDataType',{'SS_DOUBLE','SS_DOUBLE','SS_DOUBLE','SS_DOUBLE','SS_DOUBLE','SS_DOUBLE','SS_DOUBLE','SS_DOUBLE','SS_DOUBLE','SS_DOUBLE','SS_DOUBLE','SS_DOUBLE'}),'MsgIdNumFormat',0,'MsgComment',{{''}}),'Version',1.2,'general',struct('isFromLib',0)),'OFF',[]}},'GroupId',{{struct('Group',{{'RTICAN'}},'No',4,'Behavior',{{'NAMECHANGE'}},'BlockType',{{'SINK'}},'NameChangeFlag',0),'OFF',[]}},'SFcnRTICANMessage',{{struct('MsgType','RX','SFcnPortType','Scalar','MsgName','ESR_Track38','MsgIdFormat','STD','MsgId',1317,'MsgLength',8,'NumSignals',12,'SampleTime',0.01,'Signal',struct('SgnName',{'CAN_TX_TRACK_RANGE_RATE_38','CAN_TX_TRACK_MED_RANGE_MODE_38','CAN_TX_TRACK_RANGE_ACCEL_38','CAN_TX_TRACK_WIDTH_38','CAN_TX_TRACK_ROLLING_COUNT_38','CAN_TX_TRACK_BRIDGE_OBJECT_38','CAN_TX_TRACK_RANGE_38','CAN_TX_TRACK_ANGLE_38','CAN_TX_TRACK_STATUS_38','CAN_TX_TRACK_ONCOMING_38','CAN_TX_TRACK_GROUPING_CHANGED_38','CAN_TX_TRACK_LAT_RATE_38'},'SgnStartBit',{0,14,16,26,30,31,32,43,53,56,57,58},'SgnLength',{14,2,10,4,1,1,11,10,3,1,1,6},'SgnType',{'standard','standard','standard','standard','standard','standard','standard','standard','standard','standard','standard','standard'},'ModeValue',{-1,-1,-1,-1,-1,-1,-1,-1,-1,-1,-1,-1},'DataType',{['signed int'],['unsigned int'],['signed int'],['unsigned int'],['unsigned int'],['unsigned int'],['unsigned int'],['signed int'],['unsigned int'],['unsigned int'],['unsigned int'],['signed int']},'ByteLayout',{['motorola back.'],['motorola back.'],['motorola back.'],['motorola back.'],['motorola back.'],['motorola back.'],['motorola back.'],['motorola back.'],['motorola back.'],['motorola back.'],['motorola back.'],['motorola back.']},'Factor',{0.01,1,0.05,0.5,1,1,0.1,0.1,1,1,1,0.25},'Offset',{0,0,0,0,0,0,0,0,0,0,0,0},'SLDataType',{'SS_DOUBLE','SS_DOUBLE','SS_DOUBLE','SS_DOUBLE','SS_DOUBLE','SS_DOUBLE','SS_DOUBLE','SS_DOUBLE','SS_DOUBLE','SS_DOUBLE','SS_DOUBLE','SS_DOUBLE'}),'StatusSelected','no','TimeSelected','no','DeltaTimeSelected','no','BytePortSelected','no','MessageLengthSelected','no','TriggerPort',struct('Selected','no','TriggerType',0),'UserCoding',struct('Selected','no','InterfaceFile','UserDecodingFile','FcnName','UserDecodeFcn','InportSelected','no','InportWidth',1,'OutportSelected','no','OutportWidth',1),'EnablePortSelected','no','UseRXService','no','BoardType','DS1','BoardNo',2,'ControllerNo',2),'OFF',[]}},'TLCFileName',{{'rtican_rx_message','OFF',[]}})  RTISFcnParameters=struct('SFcnRTICANMessage','struct','TLCFileName','char')  RTIBlockParaDefault=struct('BoardTypeNo',4302,'BoardNo',1,'ChannelNo',1,'Parameters',struct('DataFileSupport',struct('DataFileSelectedMaster',0,'DataFileSelectedLocal',0,'DataFileName','','DataFileDate','','SelectedFile',['<no file selected>']),'Options',struct('StatusSelected',1,'TimeSelected',1,'DeltaTimeSelected',1,'BytePortSelected',0,'MessageLengthSelected',0,'TriggerPort',struct('Selected',0,'TriggerType','rising'),'UserCoding',struct('Selected',0,'InterfaceFile','UserDecodingFile','FcnName','UserDecodeFcn','InportSelected',0,'InportWidth',1,'OutportSelected',0,'OutportWidth',1),'EnablePortSelected',0,'SignalOnPortnameSelected',1,'UseRXService',0),'Message',struct('MsgOnBlocknameSelected',0,'MsgName',['RX Message'],'MsgIdFormat',0,'MsgId',100,'MsgLength',8,'NumSignals',1,'SampleTime',-1,'Signal',struct('SgnName',['RX signal'],'SgnStartBit',0,'SgnLength',8,'SgnType',0,'ModeValue',-1,'DataType',0,'SLDataType','SS_DOUBLE','ByteLayout',0,'Factor',1,'Offset',0,'Min',0,'Max',255,'SgnComment',{{}},'SgnUnit',''),'MsgIdNumFormat',0,'MsgComment',{{''}}),'Version',1.2,'general',struct('isFromLib',1)),'GroupId',struct('Group',{{'RTICAN'}},'No',1,'Behavior',{{'NAMECHANGE'}},'BlockType',{{'SINK'}},'NameChangeFlag',0),'SFcnRTICANMessage',struct('MsgType','RX','MsgName',['RX Message'],'MsgIdFormat','STD','MsgId',100,'MsgLength',8,'NumSignals',1,'SampleTime',-1,'Signal',struct('SgnName',['RX signal'],'SgnStartBit',0,'SgnLength',8,'SgnType','standard','ModeValue',-1,'DataType',['unsigned int'],'ByteLayout',['little endian'],'SLDataType','SS_DOUBLE','Factor',1,'Offset',0),'StatusSelected','yes','TimeSelected','yes','DeltaTimeSelected','yes','BytePortSelected','no','MessageLengthSelected','no','EnablePortSelected','no','UserCoding',struct('Selected','no','InterfaceFile','UserDecodingFile','FcnName','UserDecodeFcn','InportSelected','no','InportWidth',1,'OutportSelected','no','OutportWidth',1),'TriggerPort',struct('Selected','no','TriggerType','rising'),'UseRXService','no','BoardType','DS4302','BoardNo',1,'ControllerNo',1,'SFcnPortType','Scalar'),'TLCFileName','rtican_rx_message')
      settings: AttributesFormatString=Group Id: RTICAN4\n
  Out1 : Outport
  wires:
  Bus Creator/1 -> Out1/1  "Track38"
  ESR_Track38/1 -> Bus Creator/1  "CAN_TX_TRACK_RANGE_RATE_38"
  ESR_Track38/2 -> Bus Creator/2  "CAN_TX_TRACK_MED_RANGE_MODE_38"
  ESR_Track38/3 -> Bus Creator/3  "CAN_TX_TRACK_RANGE_ACCEL_38"
  ESR_Track38/4 -> Bus Creator/4  "CAN_TX_TRACK_WIDTH_38"
  ESR_Track38/5 -> Bus Creator/5  "CAN_TX_TRACK_ROLLING_COUNT_38"
  ESR_Track38/6 -> Bus Creator/6  "CAN_TX_TRACK_BRIDGE_OBJECT_38"
  ESR_Track38/7 -> Bus Creator/7  "CAN_TX_TRACK_RANGE_38"
  ESR_Track38/8 -> Bus Creator/8  "CAN_TX_TRACK_ANGLE_38"
  ESR_Track38/9 -> Bus Creator/9  "CAN_TX_TRACK_STATUS_38"
  ESR_Track38/10 -> Bus Creator/10  "CAN_TX_TRACK_ONCOMING_38"
  ESR_Track38/11 -> Bus Creator/11  "CAN_TX_TRACK_GROUPING_CHANGED_38"
  ESR_Track38/12 -> Bus Creator/12  "CAN_TX_TRACK_LAT_RATE_38"
